simulink library "dynamics"  (R2020a)
settings: Solver=VariableStepAuto  StartTime=0.0  StopTime=10.0  RelTol=1e-3
libraries: aerolibutil x1, coordinate_transforms x1, vrlib x1
settings Model: Creator=Nikita  LastModifiedBy=Nikita

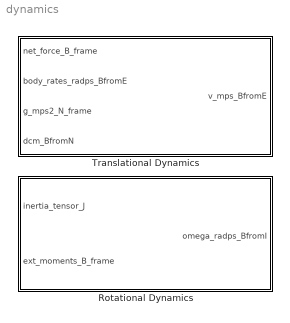
== system dynamics ==
  Rotational Dynamics : Subsystem
  Translational Dynamics : Subsystem

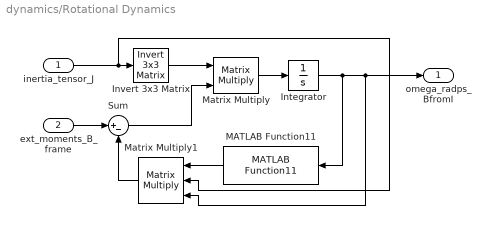
== system dynamics/Rotational Dynamics ==
  inertia_tensor_J : Inport
  ext_moments_B_frame : Inport  Port=2
  Integrator : Integrator
  Invert 3x3 Matrix : aerolibutil/Invert  3x3 Matrix
  MATLAB Function11 : coordinate_transforms/MATLAB Function11  SystemSampleTime=-1  Latency=0  AutoFrameSizeCalculation=off
  Matrix Multiply : Product  Multiplication=Matrix(*)
  Matrix Multiply1 : Product  Inputs=3  Multiplication=Matrix(*)
  Sum : Sum  Inputs=|+-
  omega_radps_BfromI : Outport
  wires:
  MATLAB Function11/1 -> Matrix Multiply1/1
  Integrator/1 -> omega_radps_BfromI/1, Matrix Multiply1/3, MATLAB Function11/1
  Matrix Multiply1/1 -> Sum/2
  Sum/1 -> Matrix Multiply/2
  Invert 3x3 Matrix/1 -> Matrix Multiply/1
  inertia_tensor_J/1 -> Matrix Multiply1/2, Invert 3x3 Matrix/1
  Matrix Multiply/1 -> Integrator/1
  ext_moments_B_frame/1 -> Sum/1

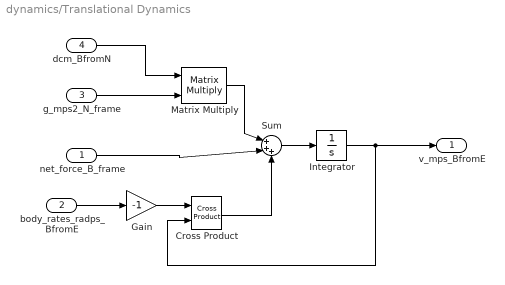
== system dynamics/Translational Dynamics ==
  net_force_B_frame : Inport
  body_rates_radps_BfromE : Inport  Port=2
  g_mps2_N_frame : Inport  Port=3
  dcm_BfromN : Inport  Port=4
  Cross Product : vrlib/Utilities/Cross Product
  Gain : Gain  Gain=-1
  Integrator : Integrator
  Matrix Multiply : Product  Multiplication=Matrix(*)
  Sum : Sum  Inputs=|+++
  v_mps_BfromE : Outport
  wires:
  net_force_B_frame/1 -> Sum/2
  Matrix Multiply/1 -> Sum/1
  Cross Product/1 -> Sum/3
  g_mps2_N_frame/1 -> Matrix Multiply/2
  dcm_BfromN/1 -> Matrix Multiply/1
  Integrator/1 -> v_mps_BfromE/1, Cross Product/2
  Sum/1 -> Integrator/1
  body_rates_radps_BfromE/1 -> Gain/1
  Gain/1 -> Cross Product/1
